simulink model "sidesplip_loop"  (Simulink 9.0)
settings: Solver=VariableStepAuto  StartTime=0.0  StopTime=30  RelTol=1e-3
InitFcn:
  | param_chap6
values from neighbouring files (symbols this model uses):
  G = getGains(P,G)    [param_chap6.m]
libraries: cstblocks x1
settings Model: SuppressorTable=22 serialization::archive 11 0 6 0 0 0 0 0  Creator=leonardopedroso  LastModifiedBy=leonardopedroso
settings DataIOCC: SaveFormat=Dataset
settings OptimizationCC: LifeSpan=auto
settings DebuggingCC: UnderspecifiedInitializationDetection=Simplified  MergeDetectMultiDrivingBlocksExec=error  SFUnexpectedBacktrackingDiag=error  SFNoUnconditionalDefaultTransitionDiag=error  SFExecutionAtInitializationDiag=warning
settings HardwareCC: ProdBitPerPointer=64  ProdBitPerSizeT=64  ProdBitPerPtrDiffT=64  ProdLargestAtomicFloat=Float  ProdIntDivRoundTo=Zero  ProdEndianess=LittleEndian  ProdWordSize=64  ProdHWDeviceType=Intel->x86-64 (Windows64)
settings ModelReferenceCC: PropagateSignalLabelsOutOfModel=on
settings CodeAppCC: StateflowObjectComments=off
settings GRTTargetCC: TargetLangStandard=C99 (ISO)
settings ConfigComp: CovMetricSettings=dwe  CovHtmlReporting=off  CovSaveCumulativeToWorkspaceVar=off  CovSaveSingleToWorkspaceVar=off  CovExternalEMLEnable=on

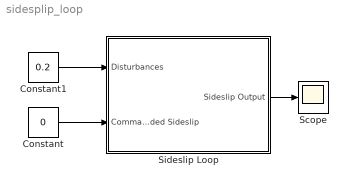
== system sidesplip_loop ==
  Constant : Constant  Value=0
  Constant1 : Constant  Value=0.2
  Scope : Scope
  "Sideslip Loop " : Subsystem
  wires:
  Constant/1 -> "Sideslip Loop "/2(Commanded Sideslip)
  "Sideslip Loop "/1(Sideslip Output) -> Scope/1
  Constant1/1 -> "Sideslip Loop "/1("Disturbances ")

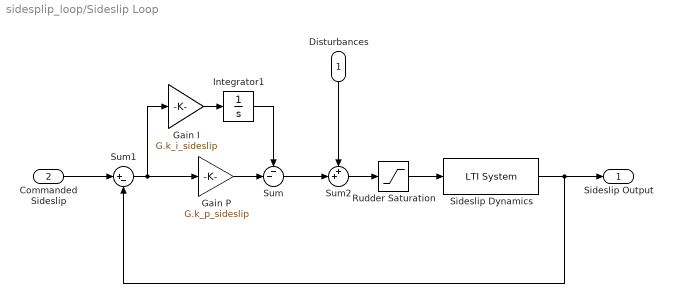
== system sidesplip_loop/Sideslip Loop  ==
  "Disturbances " : Inport
  Commanded Sideslip : Inport  Port=2
  Gain I : Gain  Gain=G.k_i_sideslip
  Gain P : Gain  Gain=G.k_p_sideslip
  Integrator1 : Integrator
  Rudder Saturation : Saturate  UpperLimit=pi/4  LowerLimit=-pi/4
  Sideslip Dynamics : cstblocks/LTI System  sys=T_v_delta_r  IC=[]
  Sum : Sum  Inputs=--|
  Sum1 : Sum  Inputs=|+-
  Sum2 : Sum  Inputs=++|
  Sideslip Output : Outport
  wires:
  Sideslip Dynamics/1 -> Sideslip Output/1, Sum1/2
  Gain P/1 -> Sum/2
  Sum1/1 -> Gain I/1, Gain P/1
  Gain I/1 -> Integrator1/1
  Integrator1/1 -> Sum/1
  Commanded Sideslip/1 -> Sum1/1
  Sum/1 -> Sum2/2
  "Disturbances "/1 -> Sum2/1
  Sum2/1 -> Rudder Saturation/1
  Rudder Saturation/1 -> Sideslip Dynamics/1
